simulink model "Cinematica_dinamica"  (R2022b)
settings: Solver=VariableStepAuto  StartTime=0.0  StopTime=10.0  RelTol=1e-3
undefined symbols (not defined in the file): d, kpR, kvL, kvR, L, lmc, LogicMap, M, R, th0, x0, y0
libraries: robotmaniplib x1, robotalgslib x1
settings Model: Creator=usuario  LastModifiedBy=usuario

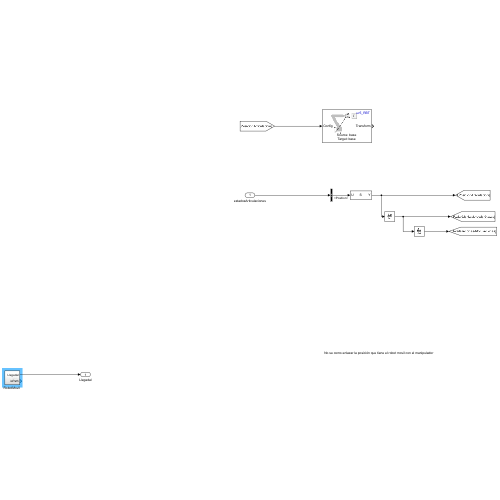
[thumbnail: Simulink's stored preview of the top-level diagram]
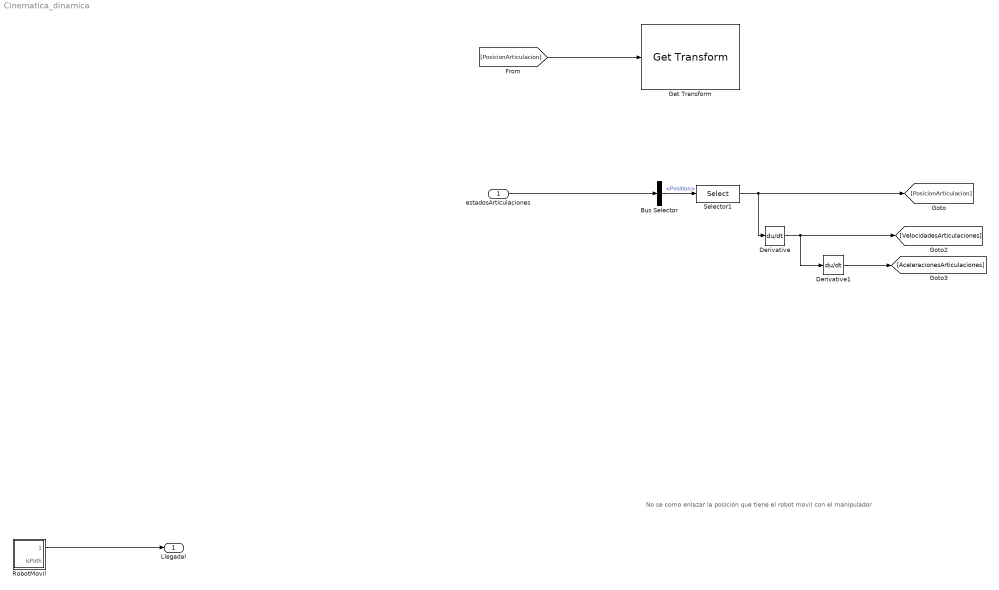
== system Cinematica_dinamica ==
  note: No se como enlazar la posición que tiene el robot movil con el manipulador
  estadosArticulaciones : Inport
  Bus Selector : BusSelector  OutputSignals=Position
  Derivative : Derivative
  Derivative1 : Derivative
  Get Transform : robotmaniplib/Get Transform  RigidBodyTree=ur5_RBT  SourceBody=base  TargetBody=base  SimulateUsing=Interpreted execution
  "RobotMovil " : Subsystem
  Selector1 : Selector  InputPortWidth=128  IndexOptions=Index vector (dialog)  Indices=[4:10]  OutputSizes=1
  Llegadal : Outport
  wires:
  Selector1/1 -> Derivative/1, [PosicionArticulacion]
  Bus Selector/1 -> Selector1/1  "<Position>"
  "RobotMovil "/1(Llegadal) -> Llegadal/1
  estadosArticulaciones/1 -> Bus Selector/1
  Derivative/1 -> [VelocidadesArticulaciones], Derivative1/1
  Derivative1/1 -> [AceleracionesArticulaciones]
  [PosicionArticulacion] -> Get Transform/1

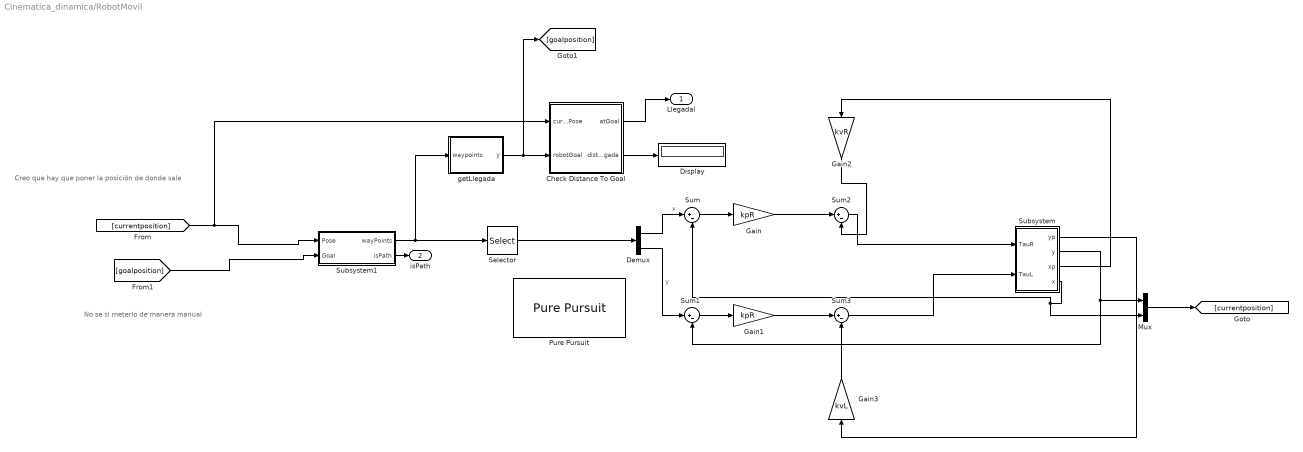
== system Cinematica_dinamica/RobotMovil  ==
  note: Creo que hay que poner la posición de donde sale
  note: No se si meterlo de manera manual
  Check Distance To Goal : Subsystem
  Demux : Demux  Outputs=2
  Display : Display
  Gain : Gain  Gain=kpR
  Gain1 : Gain  Gain=kpR
  Gain2 : Gain  Gain=kvR
  Gain3 : Gain  Gain=kvL
  Mux : Mux  Inputs=2
  Pure Pursuit : robotalgslib/Pure Pursuit  DesiredLinearVelocity=0.1  MaxAngularVelocity=1.0  LookaheadDistance=1.0  TargetDirPort=off  SimulateUsing=Code generation
      settings: LibrarySourceBlock=robotmobilelib/Pure Pursuit
  Selector : Selector  NumberOfDimensions=3  InputPortWidth=3  IndexOptions=Select all,Index vector (dialog),Index vector (dialog)  Indices=[1 2],[1 2],1  OutputSizes=1,1,1
  Subsystem : Subsystem
  Subsystem1 : Subsystem
  Sum{,1..3} (4 alike) : Sum  Inputs=|+-
  getLlegada : MATLAB Function  TreatAsAtomicUnit=on
  Llegadal : Outport
  isPath : Outport  Port=2
  wires:
  Sum1/1 -> Gain1/1
  Check Distance To Goal/1(atGoal) -> Llegadal/1
  [currentposition] -> Check Distance To Goal/1(currentPose), Subsystem1/1(Pose)
  Subsystem1/2(isPath) -> isPath/1
  getLlegada/1(y) -> [goalposition], Check Distance To Goal/2(robotGoal)
  Gain/1 -> Sum2/1
  Check Distance To Goal/2(distLlegada) -> Display/1
  Subsystem/2(y) -> Sum1/2, Mux/1
  Sum3/1 -> Subsystem/2(TauL)
  Gain3/1 -> Sum3/2
  Subsystem/3(xp) -> Gain2/1
  Sum/1 -> Gain/1
  Selector/1 -> Demux/1
  Demux/2 -> Sum1/1  "y"
  Demux/1 -> Sum/1  "x"
  Gain1/1 -> Sum3/1
  Subsystem/4(x) -> Sum/2, Mux/2
  Gain2/1 -> Sum2/2
  Sum2/1 -> Subsystem/1(TauR)
  Subsystem1/1(wayPoints) -> getLlegada/1(waypoints), Selector/1
  [goalposition] -> Subsystem1/2(Goal)
  Subsystem/1(yp) -> Gain3/1
  Mux/1 -> [currentposition]

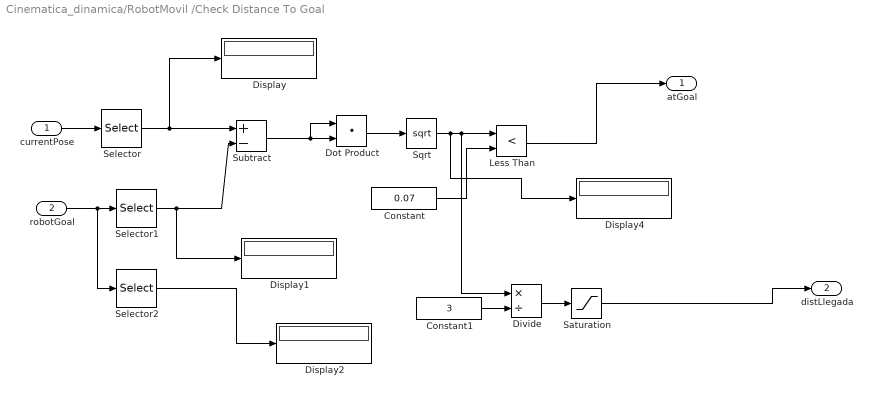
== system Cinematica_dinamica/RobotMovil /Check Distance To Goal ==
  currentPose : Inport
  robotGoal : Inport  Port=2
  Constant : Constant  Value=0.07
  Constant1 : Constant  Value=3
  Display{,1..2,4} (4 alike) : Display
  Divide : Product  Inputs=*/
  Dot Product : DotProduct  OutDataTypeStr=Inherit: Inherit via internal rule
  Less Than : RelationalOperator  Operator=<  OutDataTypeStr=boolean  RndMeth=Simplest  InputSameDT=off
  Saturation : Saturate  UpperLimit=1  LowerLimit=0.2
  Selector : Selector  InputPortWidth=3  IndexOptions=Index vector (dialog)  Indices=[1 2]  OutputSizes=1
  Selector1 : Selector  InputPortWidth=3  IndexOptions=Index vector (dialog)  Indices=[1 2]  OutputSizes=1
  Selector2 : Selector  InputPortWidth=3  IndexOptions=Index vector (dialog)  Indices=3  OutputSizes=1
  Sqrt : Sqrt
  Subtract : Sum  Inputs=+-
  atGoal : Outport
  distLlegada : Outport  Port=2
  wires:
  robotGoal/1 -> Selector2/1, Selector1/1
  Dot Product/1 -> Sqrt/1
  Constant/1 -> Less Than/2
  currentPose/1 -> Selector/1
  Sqrt/1 -> Display4/1, Divide/1, Less Than/1
  Subtract/1 -> Dot Product/1, Dot Product/2
  Selector/1 -> Display/1, Subtract/1
  Selector1/1 -> Subtract/2, Display1/1
  Selector2/1 -> Display2/1
  Less Than/1 -> atGoal/1
  Saturation/1 -> distLlegada/1
  Constant1/1 -> Divide/2
  Divide/1 -> Saturation/1

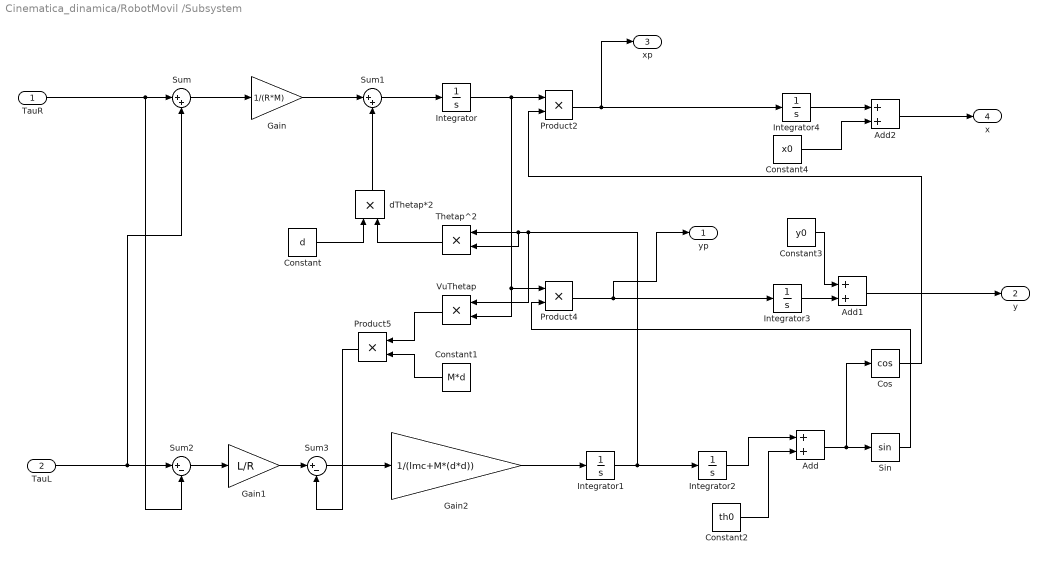
== system Cinematica_dinamica/RobotMovil /Subsystem ==
  TauR : Inport
  TauL : Inport  Port=2
  Add : Sum
  Add1 : Sum
  Add2 : Sum
  Constant : Constant  Value=d
  Constant1 : Constant  Value=M*d
  Constant2 : Constant  Value=th0
  Constant3 : Constant  Value=y0
  Constant4 : Constant  Value=x0
  Cos : Trigonometry  Operator=cos
  Gain : Gain  Gain=1/(R*M)
  Gain1 : Gain  Gain=L/R
  Gain2 : Gain  Gain=1/(lmc+M*(d*d))
  Integrator{,1..4} (5 alike) : Integrator
  Product2 : Product
  Product4 : Product
  Product5 : Product
  Sin : Trigonometry
  Sum : Sum  Inputs=|++
  Sum1 : Sum  Inputs=|++
  Sum2 : Sum  Inputs=|+-
  Sum3 : Sum  Inputs=|+-
  Thetap^2 : Product
  VuThetap : Product
  dThetap*2 : Product
  yp : Outport
  y : Outport  Port=2
  xp : Outport  Port=3
  x : Outport  Port=4
  wires:
  VuThetap/1 -> Product5/1
  Integrator1/1 -> Integrator2/1, VuThetap/1, Thetap^2/2, Thetap^2/1
  TauR/1 -> Sum2/2, Sum/1
  Product4/1 -> yp/1, Integrator3/1
  Gain1/1 -> Sum3/1
  Constant4/1 -> Add2/2
  Cos/1 -> Product2/2
  Constant2/1 -> Add/2
  Product5/1 -> Sum3/2
  Sin/1 -> Product4/2
  TauL/1 -> Sum/2, Sum2/1
  Integrator4/1 -> Add2/1
  Sum/1 -> Gain/1
  Add1/1 -> y/1
  Add/1 -> Cos/1, Sin/1
  Integrator/1 -> Product4/1, VuThetap/2, Product2/1
  Sum3/1 -> Gain2/1
  Sum2/1 -> Gain1/1
  Constant1/1 -> Product5/2
  Thetap^2/1 -> dThetap*2/2
  Gain/1 -> Sum1/1
  dThetap*2/1 -> Sum1/2
  Add2/1 -> x/1
  Constant/1 -> dThetap*2/1
  Sum1/1 -> Integrator/1
  Gain2/1 -> Integrator1/1
  Integrator2/1 -> Add/1
  Constant3/1 -> Add1/1
  Integrator3/1 -> Add1/2
  Product2/1 -> xp/1, Integrator4/1

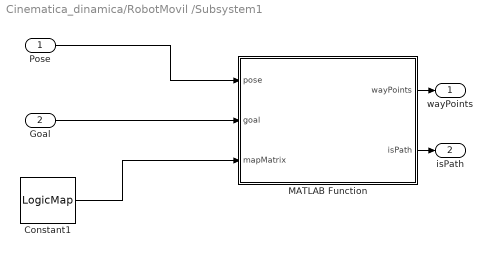
== system Cinematica_dinamica/RobotMovil /Subsystem1 ==
  Pose : Inport
  Goal : Inport  Port=2
  Constant1 : Constant  Value=LogicMap
  MATLAB Function : MATLAB Function  TreatAsAtomicUnit=on
  wayPoints : Outport
  isPath : Outport  Port=2
  wires:
  MATLAB Function/1(wayPoints) -> wayPoints/1
  Constant1/1 -> MATLAB Function/3(mapMatrix)
  Pose/1 -> MATLAB Function/1(pose)
  Goal/1 -> MATLAB Function/2(goal)
  MATLAB Function/2(isPath) -> isPath/1

== matlab function Cinematica_dinamica/RobotMovil /Subsystem1/MATLAB Function ==
  data: pose input; wayPoints output; goal input; mapMatrix input; isPath output
function [wayPoints, isPath] = plan(pose,goal,mapMatrix)


coder.extrinsic('helperPlotPathMobileArm');

ss = stateSpaceDubins; 

%Crea un mapa ocupacional basado en estados usando los state space.
binaryMap = binaryOccupancyMap(mapMatrix,10);
sv = validatorOccupancyMap(ss,"Map",binaryMap);
startPose = pose;
endPose = goal;
isPath = false;

% Comprobar si la pose inicial es lo suficientemente cerca a la goal pose
orientationDif = abs(angdiff(startPose(3), endPose(3)));
positionDif = norm(startPose(1:2)-endPose(1:2)); 

if orientationDif<=0.1 && positionDif<=0.1
    wayPoints = startPose;
    isPath = true;
    helperPlotPathMobileArm(startPose,wayPoints, mapMatrix)
    return;
end



%VALIDATION_DISTANCE
sv.ValidationDistance = 0.05;%0.01
ss.StateBounds = [binaryMap.XWorldLimits;binaryMap.YWorldLimits; [-pi pi]];
ss.MinTurningRadius = 3;%1.5;
planner = plannerRRTStar(ss,sv);
planner.MaxConnectionDistance = 0.2; 
planner.MaxNumTreeNodes = 100000;

%Estados de inicio y final
planner.MaxIterations = 100000;
planner.GoalBias = 0.5;

disp('Planning path')

rng(1); % Para un resultado repetitible
[pthObj,solnInfo] = plan(planner,startPose,endPose);
isPath = solnInfo.IsPathFound;
%Visualiza el resultado.
if isPath
    interpolate(pthObj, pthObj.NumStates * 2);
end
wayPoints = [pthObj.States;endPose]; 
helperPlotPathMobileArm(startPose,wayPoints, mapMatrix)

== matlab function Cinematica_dinamica/RobotMovil /getLlegada ==
  data: waypoints input size=[1000 3]; y output double size=[1 3]
function y = getLlegada(waypoints)
y = [0 0 0];
if ~isempty(waypoints)
    y = waypoints(end,1:3);
end
end
